simulink model "CoPT"  (R2018a)
settings: configuration reference "cs_ert" (kept outside this file)
settings Model: DataDictionary=CoPT.sldd  Creator=zhoutinglin  LastModifiedBy=zhoutinglin

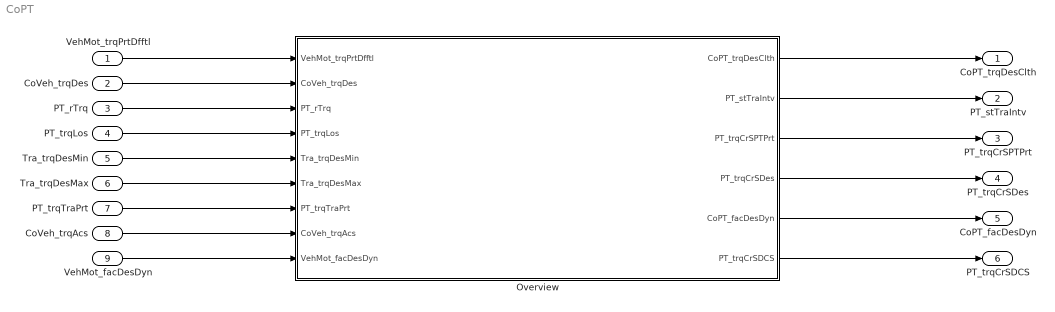
== system CoPT ==
  VehMot_trqPrtDfftl : Inport
  CoVeh_trqDes : Inport  Port=2
  PT_rTrq : Inport  Port=3
  PT_trqLos : Inport  Port=4
  Tra_trqDesMin : Inport  Port=5
  Tra_trqDesMax : Inport  Port=6
  PT_trqTraPrt : Inport  Port=7
  CoVeh_trqAcs : Inport  Port=8
  VehMot_facDesDyn : Inport  Port=9
  Overview : Subsystem
  CoPT_trqDesClth : Outport
  PT_stTraIntv : Outport  Port=2
  PT_trqCrSPTPrt : Outport  Port=3
  PT_trqCrSDes : Outport  Port=4
  CoPT_facDesDyn : Outport  Port=5
  PT_trqCrSDCS : Outport  Port=6
  wires:
  VehMot_trqPrtDfftl/1 -> Overview/1(VehMot_trqPrtDfftl)
  CoVeh_trqDes/1 -> Overview/2(CoVeh_trqDes)
  PT_rTrq/1 -> Overview/3(PT_rTrq)
  PT_trqLos/1 -> Overview/4(PT_trqLos)
  Tra_trqDesMin/1 -> Overview/5(Tra_trqDesMin)
  Tra_trqDesMax/1 -> Overview/6(Tra_trqDesMax)
  PT_trqTraPrt/1 -> Overview/7(PT_trqTraPrt)
  CoVeh_trqAcs/1 -> Overview/8(CoVeh_trqAcs)
  VehMot_facDesDyn/1 -> Overview/9(VehMot_facDesDyn)
  Overview/1(CoPT_trqDesClth) -> CoPT_trqDesClth/1
  Overview/2(PT_stTraIntv) -> PT_stTraIntv/1
  Overview/3(PT_trqCrSPTPrt) -> PT_trqCrSPTPrt/1
  Overview/4(PT_trqCrSDes) -> PT_trqCrSDes/1
  Overview/5(CoPT_facDesDyn) -> CoPT_facDesDyn/1
  Overview/6(PT_trqCrSDCS) -> PT_trqCrSDCS/1

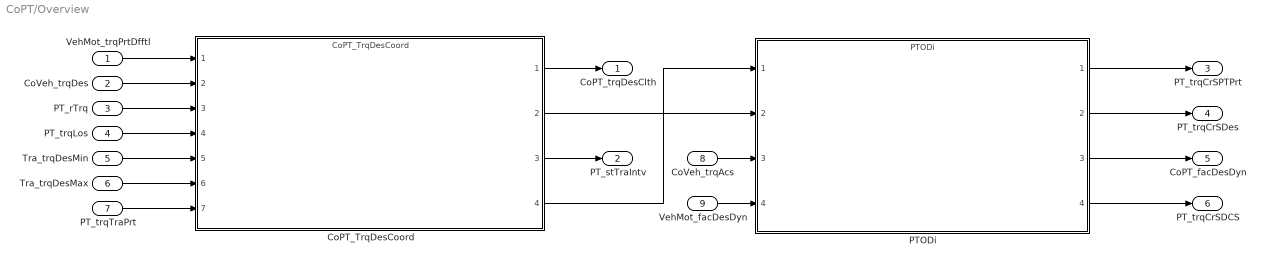
== system CoPT/Overview ==
  VehMot_trqPrtDfftl : Inport
  CoVeh_trqDes : Inport  Port=2
  PT_rTrq : Inport  Port=3
  PT_trqLos : Inport  Port=4
  Tra_trqDesMin : Inport  Port=5
  Tra_trqDesMax : Inport  Port=6
  PT_trqTraPrt : Inport  Port=7
  CoVeh_trqAcs : Inport  Port=8
  VehMot_facDesDyn : Inport  Port=9
  CoPT_TrqDesCoord : ModelReference  ModelNameDialog=CoPT_TrqDesCoord  SimulationMode=Normal  ModelReferenceVersion=1.51
  PTODi : ModelReference  ModelNameDialog=PTODi  SimulationMode=Normal  ModelReferenceVersion=1.2
  CoPT_trqDesClth : Outport
  PT_stTraIntv : Outport  Port=2
  PT_trqCrSPTPrt : Outport  Port=3
  PT_trqCrSDes : Outport  Port=4
  CoPT_facDesDyn : Outport  Port=5
  PT_trqCrSDCS : Outport  Port=6
  wires:
  CoPT_TrqDesCoord/2 -> PTODi/2
  CoPT_TrqDesCoord/4 -> PTODi/1
  VehMot_trqPrtDfftl/1 -> CoPT_TrqDesCoord/1
  CoVeh_trqDes/1 -> CoPT_TrqDesCoord/2
  PT_rTrq/1 -> CoPT_TrqDesCoord/3
  PT_trqLos/1 -> CoPT_TrqDesCoord/4
  Tra_trqDesMin/1 -> CoPT_TrqDesCoord/5
  Tra_trqDesMax/1 -> CoPT_TrqDesCoord/6
  PT_trqTraPrt/1 -> CoPT_TrqDesCoord/7
  CoPT_TrqDesCoord/1 -> CoPT_trqDesClth/1
  CoPT_TrqDesCoord/3 -> PT_stTraIntv/1
  CoVeh_trqAcs/1 -> PTODi/3
  VehMot_facDesDyn/1 -> PTODi/4
  PTODi/1 -> PT_trqCrSPTPrt/1
  PTODi/2 -> PT_trqCrSDes/1
  PTODi/3 -> CoPT_facDesDyn/1
  PTODi/4 -> PT_trqCrSDCS/1
